simulink model "oving2_oppg_q"  (R2024a)
settings: Solver=ode2  StartTime=0.0  StopTime=50  FixedStep=0.01  RelTol=1e-3
values from neighbouring files (symbols this model uses):
  Kd = 0.1    [oving2_data.m]
  Ki = 1.5    [oving2_data.m]
  Kp = 2    [oving2_data.m]
libraries: mylib x1, simulink_extras x1
settings Model: Creator=tormod  LastModifiedBy=tormod

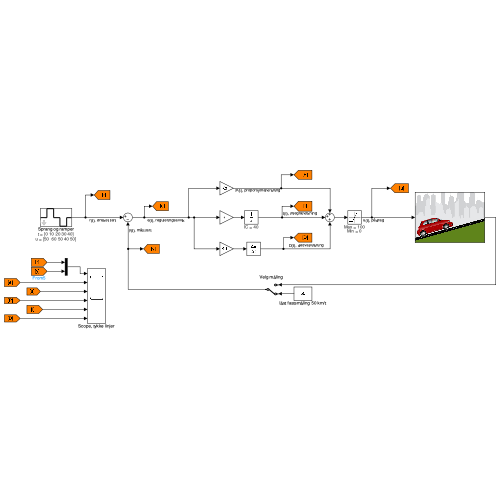
[thumbnail: Simulink's stored preview of the top-level diagram]
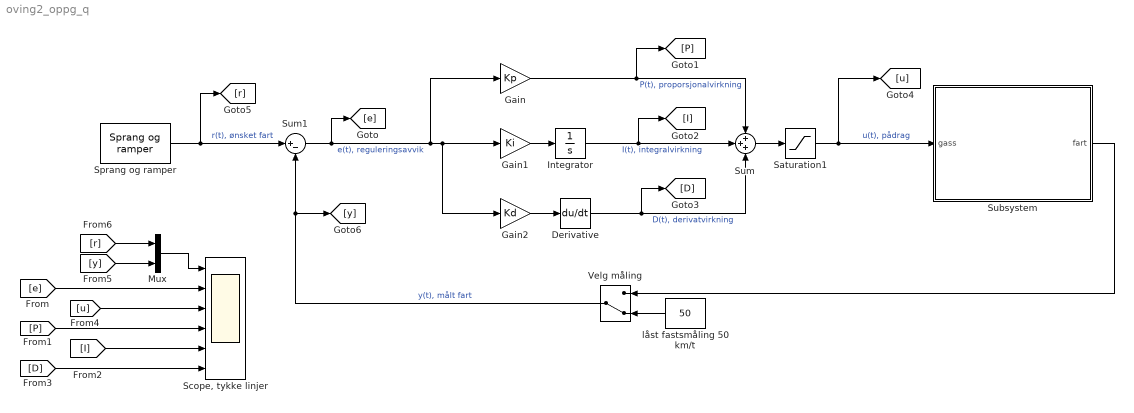
== system oving2_oppg_q ==
  Derivative : Derivative
  Gain : Gain  Gain=Kp
  Gain1 : Gain  Gain=Ki
  Gain2 : Gain  Gain=Kd
  Integrator : Integrator  InitialCondition=40  UpperSaturationLimit=100  LowerSaturationLimit=0
      settings: AttributesFormatString=IC = %<InitialCondition>
  Mux : Mux  Inputs=2
  Saturation1 : Saturate  UpperLimit=100  LowerLimit=0
      settings: AttributesFormatString=|
      | Max = %<UpperLimit>
      | Min = %<LowerLimit>
  "Scope, tykke linjer" : Scope  NumInputPorts=6
  Sprang og ramper : mylib/ELE130/Sprang og ramper  tidspunkt=[0 10 20 30 40]  utgangsverdi="[50  60 50 40 50]"  valg=Trappetrinn
      settings: SourceProductName=Eget bibliotek
      settings: AttributesFormatString=|
      | t = %<tidspunkt>
      | u = %<utgangsverdi>
  Subsystem : Subsystem
      mask Display: image('hill-start.jpg');
  Sum : Sum  Inputs=3
  Sum1 : Sum  Inputs=|+-
  Velg måling : ManualSwitch  CurrentSetting=0
  låst fastsmåling 50 km/t : Constant  Value=50
  wires:
  Sprang og ramper/1 -> [r], Sum1/1  "r(t), ønsket fart"
  Gain/1 -> [P], Sum/1  "P(t), proporsjonalvirkning"
  Sum1/1 -> Gain2/1, Gain1/1, Gain/1, [e]  "e(t), reguleringsavvik"
  Gain1/1 -> Integrator/1
  Gain2/1 -> Derivative/1
  [u] -> "Scope, tykke linjer"/3
  Velg måling/1 -> Sum1/2, [y]  "y(t), målt fart"
  Derivative/1 -> [D], Sum/3  "D(t), derivatvirkning"
  Sum/1 -> Saturation1/1
  Integrator/1 -> [I], Sum/2  "I(t), integralvirkning"
  [e] -> "Scope, tykke linjer"/2
  [D] -> "Scope, tykke linjer"/6
  låst fastsmåling 50 km/t/1 -> Velg måling/2
  [P] -> "Scope, tykke linjer"/4
  [I] -> "Scope, tykke linjer"/5
  Mux/1 -> "Scope, tykke linjer"/1
  Saturation1/1 -> Subsystem/1(gass), [u]  "u(t), pådrag"
  Subsystem/1(fart) -> Velg måling/1
  [r] -> Mux/1
  [y] -> Mux/2

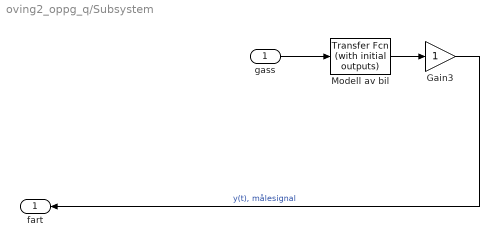
== system oving2_oppg_q/Subsystem ==
  gass : Inport
  Gain3 : Gain
  Modell av bil : simulink_extras/Additional Linear/Transfer Fcn (with initial outputs)  N=[1.25]  D="[1  1]"  Y0=50  U0=0
      settings: AttributesFormatString=Initial output %<Y0> km/t
  fart : Outport
  wires:
  Gain3/1 -> fart/1  "y(t), målesignal"
  gass/1 -> Modell av bil/1
  Modell av bil/1 -> Gain3/1
